simulink library "LinWindVel3D_ul"  (R2020a)
settings: Solver=VariableStepAuto  StartTime=0.0  StopTime=10.0  RelTol=1e-3
undefined symbols (not defined in the file): Env
settings Model: Creator=John Jr  LastModifiedBy=John Jr
settings SFSimCC: CustomCodeUndefinedFunction=UseInterfaceOnly

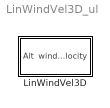
== system LinWindVel3D_ul ==
  LinWindVel3D : Subsystem
      mask DialogControl DescTextVar Prompt: This subsystem calculates the wind speed at the current input altitude. The wind speed is modeled as a linear function of altitude.
      mask Display:
      | patch([0 1 1 0], [0 0 1 1],[.8 1 1])
      | 
      | port_label('input',1,'z [m]','texmode','on')
      | 
      | port_label('output',1,'v_w [m/s]','texmode','on')

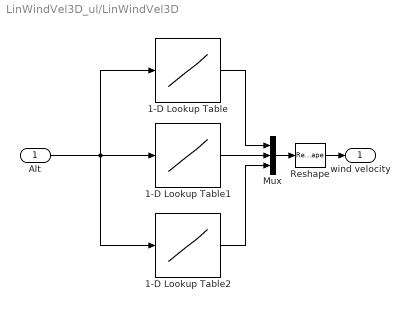
== system LinWindVel3D_ul/LinWindVel3D ==
  Alt : Inport
  1-D Lookup Table : Lookup_n-D  NumberOfTableDimensions=1  BreakpointsForDimension1=[0 5000]/3.2808  Table=Env.windVecX.Value  InternalRulePriority=Speed  RndMeth=Simplest  InputSameDT=on
  1-D Lookup Table1 : Lookup_n-D  NumberOfTableDimensions=1  BreakpointsForDimension1=[0 5000]/3.2808  Table=Env.windVecY.Value  InternalRulePriority=Speed  RndMeth=Simplest  InputSameDT=on
  1-D Lookup Table2 : Lookup_n-D  NumberOfTableDimensions=1  BreakpointsForDimension1=[0 5000]/3.2808  Table=Env.windVecZ.Value  InternalRulePriority=Speed  RndMeth=Simplest  InputSameDT=on
  Mux : Mux  Inputs=3
  Reshape : Reshape  OutputDimensionality=Column vector (2-D)
  wind velocity : Outport  VectorParamsAs1DForOutWhenUnconnected=off
  wires:
  Reshape/1 -> wind velocity/1
  Alt/1 -> 1-D Lookup Table2/1, 1-D Lookup Table/1, 1-D Lookup Table1/1
  1-D Lookup Table1/1 -> Mux/2
  Mux/1 -> Reshape/1
  1-D Lookup Table/1 -> Mux/1
  1-D Lookup Table2/1 -> Mux/3
